simulink model "L2"  (R2023a)
settings: Solver=ode45  StartTime=0.0  StopTime=10.0  RelTol=1e-3  EnableMultiTasking=on
libraries: dspinverses x1, dspsolvers x1
settings Model: Creator=autologin  LastModifiedBy=ввв
settings SolverCC: AlgebraicLoopSolver=TrustRegion
settings DataIOCC: LimitDataPoints=on  SaveFormat=Array  SignalLoggingSaveFormat=ModelDataLogs  ReturnWorkspaceOutputs=off
settings OptimizationCC: ExpressionDepthLimit=2147483647  LifeSpan=inf
settings DebuggingCC: UnderspecifiedInitializationDetection=Classic  MergeDetectMultiDrivingBlocksExec=none  SolverPrmCheckMsg=warning  FcnCallInpInsideContextMsg=warning  UnconnectedInputMsg=warning  UnconnectedOutputMsg=warning  UnconnectedLineMsg=warning  StateNameClashWarn=warning  SFUnexpectedBacktrackingDiag=warning  SFNoUnconditionalDefaultTransitionDiag=warning  SFExecutionAtInitializationDiag=none  ArithmeticOperatorsInVariantConditions=warning
settings HardwareCC: ProdBitPerPointer=32  ProdBitPerSizeT=32  ProdBitPerPtrDiffT=32  ProdLargestAtomicFloat=None  ProdIntDivRoundTo=Undefined  ProdEndianess=Unspecified  ProdWordSize=32  ProdHWDeviceType=32-bit Generic
settings ModelReferenceCC: PropagateSignalLabelsOutOfModel=off
settings SFSimCC: SimUseLocalCustomCode=off  CustomCodeUndefinedFunction=UseInterfaceOnly
settings RTWCC: RTWUseLocalCustomCode=off
settings CodeAppCC: StateflowObjectComments=on
settings GRTTargetCC: TargetLangStandard=C89/C90 (ANSI)  CombineOutputUpdateFcns=off  GRTInterface=on
settings ConfigComp: CovMetricSettings=dw  CovSaveCumulativeToWorkspaceVar=on  CovSaveSingleToWorkspaceVar=on  CovExternalEMLEnable=off

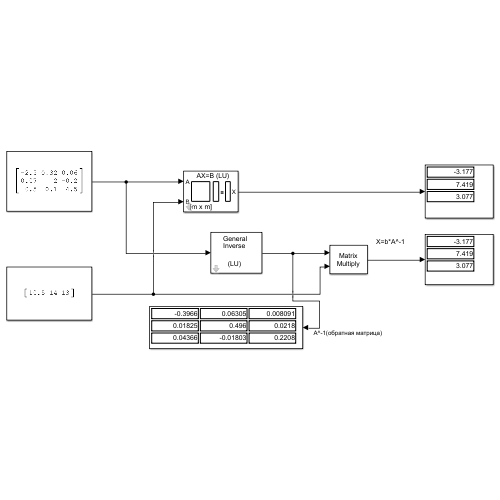
[thumbnail: Simulink's stored preview of the top-level diagram]
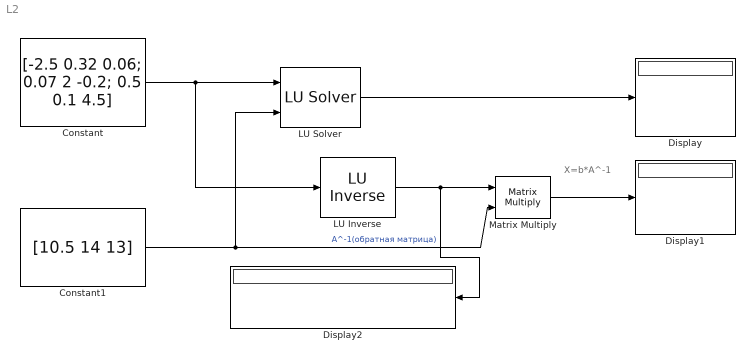
== system L2 ==
  note: X=b*A^-1
  " LU Inverse" : dspinverses/ LU Inverse
  Constant : Constant  Value=[-2.5 0.32 0.06; 0.07 2 -0.2; 0.5 0.1 4.5]
  Constant1 : Constant  Value=[10.5 14 13]
  Display : Display
  Display1 : Display
  Display2 : Display
  LU Solver : dspsolvers/LU Solver
  Matrix Multiply : Product  Multiplication=Matrix(*)
  wires:
  Constant/1 -> LU Solver/1, " LU Inverse"/1
  Matrix Multiply/1 -> Display1/1
  Constant1/1 -> Matrix Multiply/2, LU Solver/2
  " LU Inverse"/1 -> Matrix Multiply/1, Display2/1  "A^-1(обратная матрица)"
  LU Solver/1 -> Display/1
